simulink model "Control_test"  (R2014b)
settings: Solver=FixedStepDiscrete  StartTime=0.0  StopTime=Inf  FixedStep=0.001  RelTol=1e-3
PostLoadFcn:
  | , if any(exist('dsrtsu_mdlpostloadfcn', 'file') == [2, 3, 6]), try dsrtsu_mdlpostloadfcn('Execute', bdroot); catch fprintf('Error in PostLoadFcn (dsrtsu_mdlpostloadfcn) for model "%s":\n %s\n', bdroot, lasterr); end, end,
undefined symbols (not defined in the file or in its folder): dtLocal, slcm
libraries: rtican x163, simulink x14
(part 2 of 34)

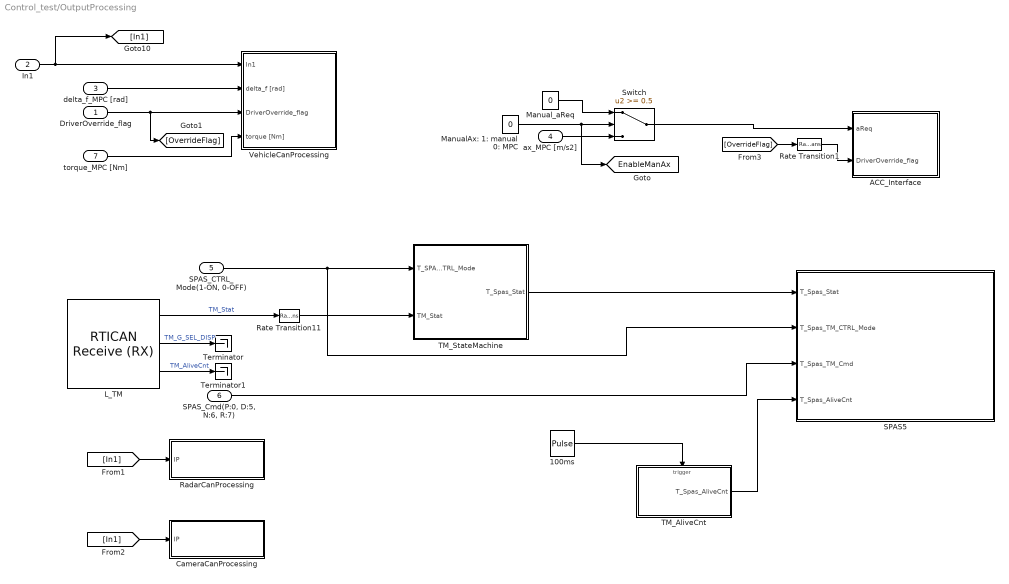
== system Control_test/OutputProcessing ==
  DriverOverride_flag : Inport
  In1 : Inport  Port=2
  delta_f_MPC [rad] : Inport  Port=3
  ax_MPC [m/s2] : Inport  Port=4
  "SPAS_CTRL_Mode(1-ON, 0-OFF)" : Inport  Port=5
  "SPAS_Cmd(P:0, D:5, N:6, R:7)" : Inport  Port=6
  torque_MPC [Nm] : Inport  Port=7
  100ms : DiscretePulseGenerator  PulseType=Time based  Period=0.1  PulseWidth=20
  ACC_Interface : Subsystem
  CameraCanProcessing : Subsystem
  L_TM : rtican/RTICAN Receive (RX)   Reserved1=[]  Reserved2=[]  Reserved3=[]  Reserved4=[]  SfcnMessage=[]  Msg_Struct=[]  BoardTypeNo=[]  BoardNo=[]  ChannelNo=[]  Parameters=[]  DialogFcn=[]  UnitName=[]  Revision=[]  UnitValues=[]  DSProperties=struct('RTI',struct('Version',uint32(5),'BlockType',struct('isSLSource',uint8(1),'isSLSink',uint8(1),'isHWSource',uint8(0),'isHWSink',uint8(0),'isSetup',uint8(0),'isInline',uint8(1),'isNonInline',uint8(0),'isInterrupt',uint8(0),'isChannelwise',uint8(0)),'IOBoardType','RTICAN','UnitType','MESSAGE','Identifier','RX','DialogType','MSVC','BlockSet','RTICAN','SlaveProcessor','CAN'))  RTIBlockInterface=struct('OutputPortsWidth',int32([1 1 1]),'OutputPortsActive',[1 1 1],'OutputPortsName',{{'TM_Stat','TM_G_SEL_DISP','TM_AliveCnt'}},'OutputPortsDataType',{{'SS_DOUBLE','SS_DOUBLE','SS_DOUBLE'}},'OutputPortsLabel',{{'TM_Stat','TM_G_SEL_DISP','TM_AliveCnt'}},'OutputPortsLabelMode','ON','InputPortsWidth',int32(0),'InputPortsActive',0,'DialogFcn','rtican_message_interface_gui','BlockDisplay',{{'','center'}},'IconTransparency','on','ParameterTunableNames',{{}},'InitLevel',3,'BlockName',struct('Token',{{'L_TM'}}),'SampleTime',{{0.1}},'TriggerPort',{{'none'}},'EnablePort',{{'none'}})  RTIBlockParameters=struct('BoardTypeNo',{{1,'OFF',[]}},'BoardNo',{{1,'ON',[1 16]}},'ChannelNo',{{1,'ON',[1 2]}},'Parameters',{{struct('DataFileSupport',struct('DataFileSelectedMaster',1,'DataFileSelectedLocal',0,'DataFileName',['e:\01_dbc_files\hmc_can_for_ucb_v2.dbc|e:\mobileye spec new\mobileye_mando_camera_ucb_v2.dbc|'],'DataFileDate',{{{['26-Nov-2014 10:54:28']},{['18-Sep-2013 10:55:24']}}},'SelectedFile',['<no file selected>'],'InterfaceFcn','rtican_dbc_file_parser'),'Options',struct('StatusSelected',0,'TimeSelected',0,'DeltaTimeSelected',0,'BytePortSelected',0,'MessageLengthSelected',0,'TriggerPort',struct('Selected',0,'TriggerType',0),'UserCoding',struct('Selected',0,'InterfaceFile','UserDecodingFile','FcnName','UserDecodeFcn','InportSelected',0,'InportWidth',1,'OutportSelected',0,'OutportWidth',1),'EnablePortSelected',0,'SignalOnPortnameSelected',1,'UseRXService',0),'Message',struct('MsgOnBlocknameSelected',1,'MsgName','L_TM','MsgIdFormat',0,'MsgId',1585,'MsgLength',8,'NumSignals',3,'SampleTime',0.1,'Signal',struct('SgnName',{'TM_Stat','TM_G_SEL_DISP','TM_AliveCnt'},'SgnStartBit',{0,8,16},'SgnLength',{4,4,4},'SgnType',{0,0,0},'ModeValue',{-1,-1,-1},'DataType',{1,1,0},'ByteLayout',{0,0,0},'Factor',{1,1,1},'Offset',{0,0,0},'SgnComment',{{''},{''},{''}},'SgnUnit',{'','',''},'Min',{0,0,0},'Max',{0,0,0},'SLDataType',{'SS_DOUBLE','SS_DOUBLE','SS_DOUBLE'}),'MsgIdNumFormat',0,'MsgComment',{{''}}),'Version',1.2,'general',struct('isFromLib',0)),'OFF',[]}},'GroupId',{{struct('Group',{{'RTICAN'}},'No',1,'Behavior',{{'NAMECHANGE'}},'BlockType',{{'SINK'}},'NameChangeFlag',0),'OFF',[]}},'SFcnRTICANMessage',{{struct('MsgType','RX','SFcnPortType','Scalar','MsgName','L_TM','MsgIdFormat','STD','MsgId',1585,'MsgLength',8,'NumSignals',3,'SampleTime',0.1,'Signal',struct('SgnName',{'TM_Stat','TM_G_SEL_DISP','TM_AliveCnt'},'SgnStartBit',{0,8,16},'SgnLength',{4,4,4},'SgnType',{'standard','standard','standard'},'ModeValue',{-1,-1,-1},'DataType',{['signed int'],['signed int'],['unsigned int']},'ByteLayout',{['little endian'],['little endian'],['little endian']},'Factor',{1,1,1},'Offset',{0,0,0},'SLDataType',{'SS_DOUBLE','SS_DOUBLE','SS_DOUBLE'}),'StatusSelected','no','TimeSelected','no','DeltaTimeSelected','no','BytePortSelected','no','MessageLengthSelected','no','TriggerPort',struct('Selected','no','TriggerType',0),'UserCoding',struct('Selected','no','InterfaceFile','UserDecodingFile','FcnName','UserDecodeFcn','InportSelected','no','InportWidth',1,'OutportSelected','no','OutportWidth',1),'EnablePortSelected','no','UseRXService','no','BoardType','DS1','BoardNo',1,'ControllerNo',1),'OFF',[]}},'TLCFileName',{{'rtican_rx_message','OFF',[]}})  RTISFcnParameters=struct('SFcnRTICANMessage','struct','TLCFileName','char')  RTIBlockParaDefault=struct('BoardTypeNo',4302,'BoardNo',1,'ChannelNo',1,'Parameters',struct('DataFileSupport',struct('DataFileSelectedMaster',0,'DataFileSelectedLocal',0,'DataFileName','','DataFileDate','','SelectedFile',['<no file selected>']),'Options',struct('StatusSelected',1,'TimeSelected',1,'DeltaTimeSelected',1,'BytePortSelected',0,'MessageLengthSelected',0,'TriggerPort',struct('Selected',0,'TriggerType','rising'),'UserCoding',struct('Selected',0,'InterfaceFile','UserDecodingFile','FcnName','UserDecodeFcn','InportSelected',0,'InportWidth',1,'OutportSelected',0,'OutportWidth',1),'EnablePortSelected',0,'SignalOnPortnameSelected',1,'UseRXService',0),'Message',struct('MsgOnBlocknameSelected',0,'MsgName',['RX Message'],'MsgIdFormat',0,'MsgId',100,'MsgLength',8,'NumSignals',1,'SampleTime',-1,'Signal',struct('SgnName',['RX signal'],'SgnStartBit',0,'SgnLength',8,'SgnType',0,'ModeValue',-1,'DataType',0,'SLDataType','SS_DOUBLE','ByteLayout',0,'Factor',1,'Offset',0,'Min',0,'Max',255,'SgnComment',{{}},'SgnUnit',''),'MsgIdNumFormat',0,'MsgComment',{{''}}),'Version',1.2,'general',struct('isFromLib',1)),'GroupId',struct('Group',{{'RTICAN'}},'No',1,'Behavior',{{'NAMECHANGE'}},'BlockType',{{'SINK'}},'NameChangeFlag',0),'SFcnRTICANMessage',struct('MsgType','RX','MsgName',['RX Message'],'MsgIdFormat','STD','MsgId',100,'MsgLength',8,'NumSignals',1,'SampleTime',-1,'Signal',struct('SgnName',['RX signal'],'SgnStartBit',0,'SgnLength',8,'SgnType','standard','ModeValue',-1,'DataType',['unsigned int'],'ByteLayout',['little endian'],'SLDataType','SS_DOUBLE','Factor',1,'Offset',0),'StatusSelected','yes','TimeSelected','yes','DeltaTimeSelected','yes','BytePortSelected','no','MessageLengthSelected','no','EnablePortSelected','no','UserCoding',struct('Selected','no','InterfaceFile','UserDecodingFile','FcnName','UserDecodeFcn','InportSelected','no','InportWidth',1,'OutportSelected','no','OutportWidth',1),'TriggerPort',struct('Selected','no','TriggerType','rising'),'UseRXService','no','BoardType','DS4302','BoardNo',1,'ControllerNo',1,'SFcnPortType','Scalar'),'TLCFileName','rtican_rx_message')
      settings: AttributesFormatString=Group Id: RTICAN1\n
  ManualAx: 1: manual 0: MPC : Constant  Value=0
  Manual_aReq : Constant  Value=0
  RadarCanProcessing : Subsystem
  Rate Transition1 : RateTransition  OutPortSampleTime=0.02
  Rate Transition11 : RateTransition  OutPortSampleTime=0.1
  SPAS5 : Subsystem
  Switch : Switch  Threshold=0.5
  TM_AliveCnt : Subsystem
  TM_StateMachine : Stateflow chart  TreatAsAtomicUnit=on
  Terminator : Terminator
  Terminator1 : Terminator
  VehicleCanProcessing : Subsystem
  tag scope: EnableManAx=global
  wires:
  delta_f_MPC [rad]/1 -> VehicleCanProcessing/2(delta_f [rad])
  Manual_aReq/1 -> Switch/1
  ManualAx: 1: manual 0: MPC/1 -> [EnableManAx], Switch/2
  ax_MPC [m/s2]/1 -> Switch/3
  Switch/1 -> ACC_Interface/1(aReq)
  DriverOverride_flag/1 -> [OverrideFlag], VehicleCanProcessing/3(DriverOverride_flag)
  Rate Transition1/1 -> ACC_Interface/2(DriverOverride_flag)
  TM_StateMachine/1(T_Spas_Stat) -> SPAS5/1(T_Spas_Stat)
  "SPAS_Cmd(P:0, D:5, N:6, R:7)"/1 -> SPAS5/3(T_Spas_TM_Cmd)
  L_TM/1 -> Rate Transition11/1  "TM_Stat"
  "SPAS_CTRL_Mode(1-ON, 0-OFF)"/1 -> TM_StateMachine/1(T_SPAS_TM_CTRL_Mode), SPAS5/2(T_Spas_TM_CTRL_Mode)
  100ms/1 -> TM_AliveCnt/Trigger
  TM_AliveCnt/1(T_Spas_AliveCnt) -> SPAS5/4(T_Spas_AliveCnt)
  Rate Transition11/1 -> TM_StateMachine/2(TM_Stat)
  L_TM/3 -> Terminator1/1  "TM_AliveCnt"
  L_TM/2 -> Terminator/1  "TM_G_SEL_DISP"
  In1/1 -> [In1], VehicleCanProcessing/1(In1)
  [In1] -> RadarCanProcessing/1(IP)
  [In1] -> CameraCanProcessing/1(IP)
  [OverrideFlag] -> Rate Transition1/1
  torque_MPC [Nm]/1 -> VehicleCanProcessing/4(torque [Nm])

== system Control_test/RTI Data ==
  RTI Data Store : Subsystem  Tag="struct('public',struct('sub',struct('name',{{'Control_test'}},'data',{{struct('TH',struct('thTaskInfo',struct('taskType',{'TIMER','HWINT','TMRINT','SWINT','GLINT'},'tasksNumOf',{5,0,0,0,0},'srcIds',{{'TIMERA','TIMERA2','TIMERA3','TIMERA4','TIMERA5'},{},{},{},{}},'taskNames',{{['Timer Task 1'],['Timer Task 2'],['Timer Task 3'],['Timer Task 4'],['Timer Task 5']},{},{},{},{}})),'th_tc',struct('dataType',{'TASK','TASK','TASK','TASK','TASK'},'taskGroupId',{'','','','',''},'taskGroupList',{{},{},{},{},{}},'taskSchedulingPolicy',{'FCFS','FCFS','FCFS','FCFS','FCFS'},'taskType',{'TIMER','TIMER','TIMER','TIMER','TIMER'},'blkh',{-1,-1,-1,-1,-1},'srcId',{'TIMERA','TIMERA2','TIMERA3','TIMERA4','TIMERA5'},'srcSgnName',{['Timer A interrupt'],['Timer Task 1'],['Timer Task 1'],['Timer Task 1'],['Timer Task 1']},'srcCpuName',{'','','','',''},'taskName',{['Timer Task 1  [0.001] s'],['Timer Task 2  [0.01] s'],['Timer Task 3  [0.02] s'],['Timer Task 4  [0.05] s'],['Timer Task 5  [0.1] s']},'taskNameDisplayExt',{'','','','',''},'smplTime',{0.001,0.01,0.02,0.05,0.1},'smplTimeOffs',{0,0,0,0,0},'hasFixedPriority',{0,0,0,0,0},'priority',{1,2,3,4,5},'hasFixedOvc',{0,0,0,0,0},'ovcType',{1,1,1,1,1},'ovcMax',{1,1,1,1,1}),'tc_th',struct('dataType',{'TASK','TASK','TASK','TASK','TASK'},'taskGroupId',{'','','','',''},'taskGroupList',{{},{},{},{},{}},'taskSchedulingPolicy',{'FCFS','FCFS','FCFS','FCFS','FCFS'},'taskType',{'TIMER','TIMER','TIMER','TIMER','TIMER'},'blkh',{-1,-1,-1,-1,-1},'srcId',{'TIMERA','TIMERA2','TIMERA3','TIMERA4','TIMERA5'},'srcSgnName',{['Timer A interrupt'],['Timer Task 1'],['Timer Task 1'],['Timer Task 1'],['Timer Task 1']},'srcCpuName',{'','','','',''},'taskName',{['Timer Task 1  [0.001] s'],['Timer Task 2  [0.01] s'],['Timer Task 3  [0.02] s'],['Timer Task 4  [0.05] s'],['Timer Task 5  [0.1] s']},'taskNameDisplayExt',{'','','','',''},'smplTime',{0.001,0.01,0.02,0.05,0.1},'smplTimeOffs',{0,0,0,0,0},'hasFixedPriority',{0,0,0,0,0},'priority',{1,2,3,4,5},'hasFixedOvc',{0,0,0,0,0},'ovcType',{1,1,1,1,1},'ovcMax',{1,1,1,1,1}))}})),'private',struct('version',struct('dsVer',uint32(2)),'access',struct('modified',['07-Mar-2016 10:47:59'],'type','Model','isPerm',1)))"  mask(RTI_DATA_STORE){}
      mask help:
      | RTI Data Store Block. This block is used by RTI to store internal model dependent data. Deleting this block will result in data loss.
      |
      | NEVER DELETE, COPY, OR MODIFY THIS BLOCK!
      mask Help:
      | RTI Data Store Block. This block is used by RTI to store internal model dependent data. Deleting this block will result in data loss.
      | 
      | NEVER DELETE, COPY, OR MODIFY THIS BLOCK!
      mask Display: text(0.5, 0.5, ' ', 'HorizontalAlignment', 'center');

== system Control_test/SensorFusion ==
  In1 : Inport
  Map-based Localization : Subsystem  SystemSampleTime=dtLocal
  OutMap : Outport
  wires:
  In1/1 -> Map-based Localization/1(In1)
  Map-based Localization/1(OutMap) -> OutMap/1

== system Control_test/Controller/CalBelief Subsystem ==
  sigma : Inport
  b_q : Inport  Port=2
  x_next : Inport  Port=3  PortDimensions=4
  xk : Inport  Port=4  PortDimensions=4
  reactiveDist : Inport  Port=5
  safeDist : Inport  Port=6
  MATLAB Function1 : MATLAB Function  TreatAsAtomicUnit=on
  b_x_next : Outport  PortDimensions=4
  b_q_next : Outport  Port=2  PortDimensions=12
  wires:
  reactiveDist/1 -> MATLAB Function1/5(reactiveDist)
  b_q/1 -> MATLAB Function1/1(b_q)
  xk/1 -> MATLAB Function1/2(xk)
  sigma/1 -> MATLAB Function1/4(sigma)
  MATLAB Function1/2(b_x_next) -> b_x_next/1
  safeDist/1 -> MATLAB Function1/6(safeDist)
  x_next/1 -> MATLAB Function1/3(x_next)
  MATLAB Function1/1(b_q_next) -> b_q_next/1

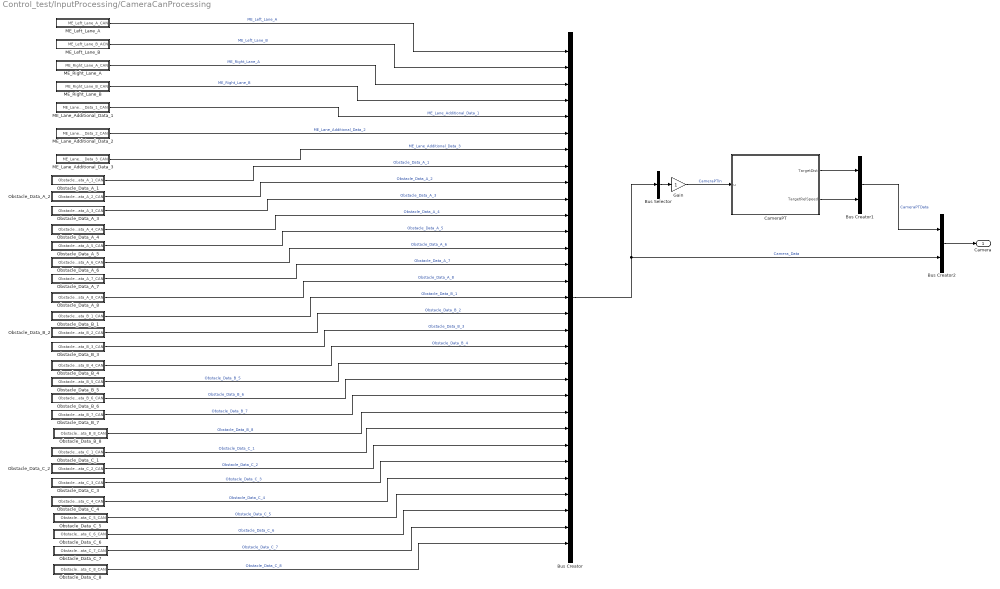
== system Control_test/InputProcessing/CameraCanProcessing ==
  Bus Creator : BusCreator  Inputs=31
  Bus Creator1 : BusCreator  Inputs=2
  Bus Creator2 : BusCreator  Inputs=2
  Bus Selector : BusSelector  OutputSignals=Obstacle_Data_A_1.CIPV_A_1,Obstacle_Data_A_2.CIPV_A_2,Obstacle_Data_A_3.CIPV_A_3,Obstacle_Data_A_4.CIPV_A_4,Obstacle_Data_A_5.CIPV_A_5,Obstacle_Data_A_6.CIPV_A_6,Obstacle_Data_A_7.CIPV_A_7,Obstacle_Data_A_8.CIPV_A_8,Obstacle_Data_B_1.Range_B_1,Obstacle_Data_B_2.Range_B_2,Obstacle_Data_B_3.Range_B_3,Obstacle_Data_B_4.Range_B_4,Obstacle_Data_B_5.Range_B_5,Obstacle_Data_B_6.Range_B_6,Obstacle_Data_B_7.Range_B_7,Obstacle_Data_B_8.Range_B_8,Obstacle_Data_B_1.RangeRate_B_1,Obstacle_Data_B_2.RangeRate_B_2,Obstacle_Data_B_3.RangeRate_B_3,Obstacle_Data_B_4.RangeRate_B_4,Obstacle_Data_B_5.RangeRate_B_5,Obstacle_Data_B_6.RangeRate_B_6,Obstacle_Data_B_7.RangeRate_B_7,Obstacle_Data_B_8.RangeRate_B_8  OutputAsBus=on
  CameraPT : MATLAB Function  TreatAsAtomicUnit=on
  Gain : Gain
  ME_Lane_Additional_Data_1 : Subsystem
  ME_Lane_Additional_Data_2 : Subsystem
  ME_Lane_Additional_Data_3 : Subsystem
  ME_Left_Lane_A : Subsystem
  ME_Left_Lane_B : Subsystem
  ME_Right_Lane_A : Subsystem
  ME_Right_Lane_B : Subsystem
  Obstacle_Data_A_1 : Subsystem
  Obstacle_Data_A_2 : Subsystem
  Obstacle_Data_A_3 : Subsystem
  Obstacle_Data_A_4 : Subsystem
  Obstacle_Data_A_5 : Subsystem
  Obstacle_Data_A_6 : Subsystem
  Obstacle_Data_A_7 : Subsystem
  Obstacle_Data_A_8 : Subsystem
  Obstacle_Data_B_1 : Subsystem
  Obstacle_Data_B_2 : Subsystem
  Obstacle_Data_B_3 : Subsystem
  Obstacle_Data_B_4 : Subsystem
  Obstacle_Data_B_5 : Subsystem
  Obstacle_Data_B_6 : Subsystem
  Obstacle_Data_B_7 : Subsystem
  Obstacle_Data_B_8 : Subsystem
  Obstacle_Data_C_1 : Subsystem
  Obstacle_Data_C_2 : Subsystem
  Obstacle_Data_C_3 : Subsystem
  Obstacle_Data_C_4 : Subsystem
  Obstacle_Data_C_5 : Subsystem
  Obstacle_Data_C_6 : Subsystem
  Obstacle_Data_C_7 : Subsystem
  Obstacle_Data_C_8 : Subsystem
  Camera : Outport
  wires:
  Bus Creator/1 -> Bus Selector/1, Bus Creator2/2  "Camera_Data"
  ME_Left_Lane_A/1(ME_Left_Lane_A_CAN) -> Bus Creator/1  "ME_Left_Lane_A"
  ME_Left_Lane_B/1(ME_Left_Lane_B_ACN) -> Bus Creator/2  "ME_Left_Lane_B"
  ME_Right_Lane_A/1(ME_Right_Lane_A_CAN) -> Bus Creator/3  "ME_Right_Lane_A"
  ME_Right_Lane_B/1(ME_Right_Lane_B_CAN) -> Bus Creator/4  "ME_Right_Lane_B"
  ME_Lane_Additional_Data_1/1(ME_Lane_Additional_Data_1_CAN) -> Bus Creator/5  "ME_Lane_Additional_Data_1"
  ME_Lane_Additional_Data_2/1(ME_Lane_Additional_Data_2_CAN) -> Bus Creator/6  "ME_Lane_Additional_Data_2"
  ME_Lane_Additional_Data_3/1(ME_Lane_Additional_Data_3_CAN) -> Bus Creator/7  "ME_Lane_Additional_Data_3"
  Obstacle_Data_A_1/1(Obstacle_Data_A_1_CAN) -> Bus Creator/8  "Obstacle_Data_A_1"
  Obstacle_Data_A_2/1(Obstacle_Data_A_2_CAN) -> Bus Creator/9  "Obstacle_Data_A_2"
  Obstacle_Data_A_3/1(Obstacle_Data_A_3_CAN) -> Bus Creator/10  "Obstacle_Data_A_3"
  Obstacle_Data_A_4/1(Obstacle_Data_A_4_CAN) -> Bus Creator/11  "Obstacle_Data_A_4"
  Obstacle_Data_A_5/1(Obstacle_Data_A_5_CAN) -> Bus Creator/12  "Obstacle_Data_A_5"
  Obstacle_Data_A_6/1(Obstacle_Data_A_6_CAN) -> Bus Creator/13  "Obstacle_Data_A_6"
  Obstacle_Data_A_7/1(Obstacle_Data_A_7_CAN) -> Bus Creator/14  "Obstacle_Data_A_7"
  Obstacle_Data_A_8/1(Obstacle_Data_A_8_CAN) -> Bus Creator/15  "Obstacle_Data_A_8"
  Obstacle_Data_B_1/1(Obstacle_Data_B_1_CAN) -> Bus Creator/16  "Obstacle_Data_B_1"
  Obstacle_Data_B_2/1(Obstacle_Data_B_2_CAN) -> Bus Creator/17  "Obstacle_Data_B_2"
  Obstacle_Data_B_3/1(Obstacle_Data_B_3_CAN) -> Bus Creator/18  "Obstacle_Data_B_3"
  Obstacle_Data_B_4/1(Obstacle_Data_B_4_CAN) -> Bus Creator/19  "Obstacle_Data_B_4"
  Obstacle_Data_B_5/1(Obstacle_Data_B_5_CAN) -> Bus Creator/20  "Obstacle_Data_B_5"
  Obstacle_Data_B_6/1(Obstacle_Data_B_6_CAN) -> Bus Creator/21  "Obstacle_Data_B_6"
  Obstacle_Data_B_7/1(Obstacle_Data_B_7_CAN) -> Bus Creator/22  "Obstacle_Data_B_7"
  Obstacle_Data_B_8/1(Obstacle_Data_B_8_CAN) -> Bus Creator/23  "Obstacle_Data_B_8"
  Obstacle_Data_C_1/1(Obstacle_Data_C_1_CAN) -> Bus Creator/24  "Obstacle_Data_C_1"
  Obstacle_Data_C_2/1(Obstacle_Data_C_2_CAN) -> Bus Creator/25  "Obstacle_Data_C_2"
  Obstacle_Data_C_3/1(Obstacle_Data_C_3_CAN) -> Bus Creator/26  "Obstacle_Data_C_3"
  Obstacle_Data_C_4/1(Obstacle_Data_C_4_CAN) -> Bus Creator/27  "Obstacle_Data_C_4"
  Obstacle_Data_C_5/1(Obstacle_Data_C_5_CAN) -> Bus Creator/28  "Obstacle_Data_C_5"
  Obstacle_Data_C_6/1(Obstacle_Data_C_6_CAN) -> Bus Creator/29  "Obstacle_Data_C_6"
  Obstacle_Data_C_7/1(Obstacle_Data_C_7_CAN) -> Bus Creator/30  "Obstacle_Data_C_7"
  Obstacle_Data_C_8/1(Obstacle_Data_C_8_CAN) -> Bus Creator/31  "Obstacle_Data_C_8"
  Bus Selector/1 -> Gain/1
  CameraPT/1(TargetDist) -> Bus Creator1/1
  CameraPT/2(TargetRelSpeed) -> Bus Creator1/2
  Bus Creator2/1 -> Camera/1
  Bus Creator1/1 -> Bus Creator2/1  "CameraPTData"
  Gain/1 -> CameraPT/1(u)  "CameraPTIn"
